simulink model "puma560_simulink"  (R2015a)
settings: Solver=ode45  StartTime=0.0  StopTime=10  MaxStep=Ts  RelTol=1e-6  AbsTol=1e-6
values from neighbouring files (symbols this model uses):
  Ts = 0.001    [bodediagram_0.m]    (also in bodediagram_1.m = 0.0005)
libraries: robotlib x11, simulink x3
settings Model: Creator=jwcjdenissen  LastModifiedBy=jwcjdenissen
settings DataIOCC: LimitDataPoints=off  SaveOutput=off  SaveTime=off
settings DebuggingCC: UnconnectedInputMsg=none  UnconnectedOutputMsg=none  UnconnectedLineMsg=none

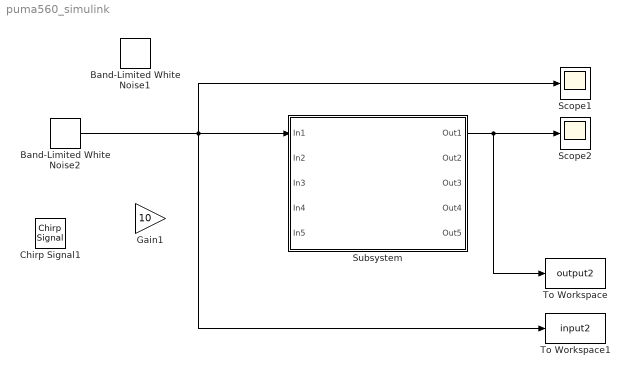
== system puma560_simulink ==
  Band-Limited White Noise1 : simulink/Sources/Band-Limited White Noise  Cov=[0.1]  Ts=Ts  seed=[round(rand*10000)]
  Band-Limited White Noise2 : simulink/Sources/Band-Limited White Noise  Cov=[0.1]  Ts=Ts  seed=[round(rand*10000)]
  Chirp Signal1 : simulink/Sources/Chirp Signal  f1=0.01  T=10  f2=100
  Gain1 : Gain  Gain=10
  Scope1 : Scope
      settings: TimeRange=1.600000000000001  YMin=-22.5  YMax=25
  Scope2 : Scope
      settings: TimeRange=2  YMin=-0.725  YMax=-0.525  SaveName=ScopeData2
  Subsystem : Subsystem
  To Workspace : ToWorkspace  VariableName=output2  SaveFormat=Timeseries  SampleTime=-1
  To Workspace1 : ToWorkspace  VariableName=input2  SaveFormat=Timeseries  SampleTime=-1
  wires:
  Subsystem/1(Out1) -> Scope2/1, To Workspace/1
  Band-Limited White Noise2/1 -> Scope1/1, To Workspace1/1, Subsystem/1(In1)

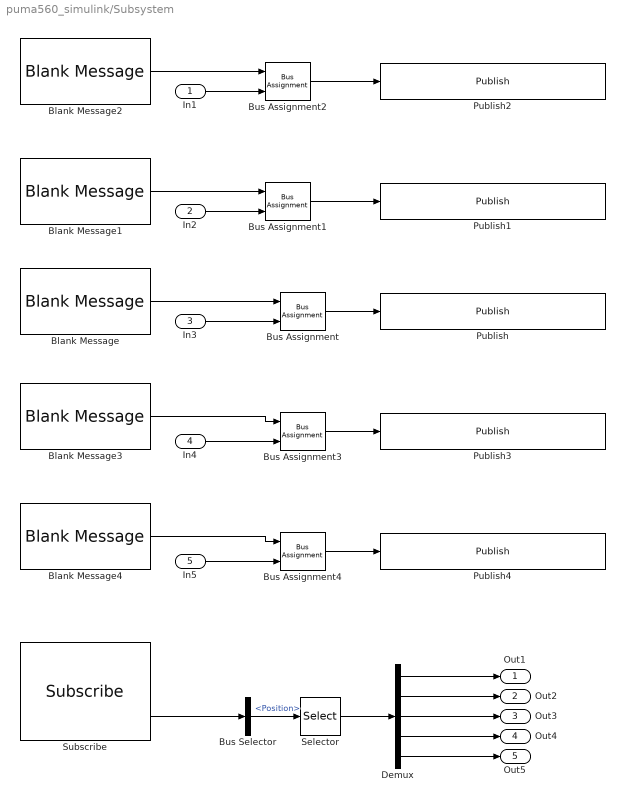
== system puma560_simulink/Subsystem ==
  In1 : Inport
  In2 : Inport  Port=2
  In3 : Inport  Port=3
  In4 : Inport  Port=4
  In5 : Inport  Port=5
  Blank Message{,1..4} (5 alike) : robotlib/Blank Message  SourceLibraryInfo=This block requires Robotics System Toolbox  messageType=std_msgs/Float64  SampleTime=inf
  Bus Assignment{,1..4} (5 alike) : BusAssignment  AssignedSignals=Data
  Bus Selector : BusSelector  OutputSignals=Position
  Demux : Demux  Outputs=5
  Publish : robotlib/Publish  SourceLibraryInfo=This block requires Robotics System Toolbox  topicSource=Specify your own  topic=/puma560/joint_3_effort_controller/command  messageType=std_msgs/Float64  messageQueueLength=1
  Publish1 : robotlib/Publish  SourceLibraryInfo=This block requires Robotics System Toolbox  topicSource=Specify your own  topic=/puma560/joint_2_effort_controller/command  messageType=std_msgs/Float64  messageQueueLength=1
  Publish2 : robotlib/Publish  SourceLibraryInfo=This block requires Robotics System Toolbox  topicSource=Specify your own  topic=/puma560/joint_1_effort_controller/command  messageType=std_msgs/Float64  messageQueueLength=1
  Publish3 : robotlib/Publish  SourceLibraryInfo=This block requires Robotics System Toolbox  topicSource=Specify your own  topic=/puma560/joint_4_effort_controller/command  messageType=std_msgs/Float64  messageQueueLength=1
  Publish4 : robotlib/Publish  SourceLibraryInfo=This block requires Robotics System Toolbox  topicSource=Specify your own  topic=/puma560/joint_5_effort_controller/command  messageType=std_msgs/Float64  messageQueueLength=1
  Selector : Selector  InputPortWidth=128  Indices=[1 2 3 4 5]
  Subscribe : robotlib/Subscribe  SourceLibraryInfo=This block requires Robotics System Toolbox  topicSource=Specify your own  topic=/puma560/joint_states  messageType=sensor_msgs/JointState  sampleTime=-1  messageQueueLength=1
  Out1 : Outport
  Out2 : Outport  Port=2
  Out3 : Outport  Port=3
  Out4 : Outport  Port=4
  Out5 : Outport  Port=5
  wires:
  Blank Message/1 -> Bus Assignment/1
  Bus Assignment/1 -> Publish/1
  Blank Message1/1 -> Bus Assignment1/1
  Bus Assignment1/1 -> Publish1/1
  Blank Message2/1 -> Bus Assignment2/1
  Bus Assignment2/1 -> Publish2/1
  Blank Message3/1 -> Bus Assignment3/1
  Bus Assignment3/1 -> Publish3/1
  Blank Message4/1 -> Bus Assignment4/1
  Bus Assignment4/1 -> Publish4/1
  In1/1 -> Bus Assignment2/2
  In3/1 -> Bus Assignment/2
  In4/1 -> Bus Assignment3/2
  In5/1 -> Bus Assignment4/2
  In2/1 -> Bus Assignment1/2
  Subscribe/2 -> Bus Selector/1
  Bus Selector/1 -> Selector/1  "<Position>"
  Selector/1 -> Demux/1
  Demux/1 -> Out1/1
  Demux/5 -> Out5/1
  Demux/4 -> Out4/1
  Demux/3 -> Out3/1
  Demux/2 -> Out2/1
